simulink model "reg_3_model"  (R2019b)
settings: Solver=VariableStepAuto  StartTime=reg3.ti  StopTime=inf  MaxStep=1e-4  RelTol=1e-9
undefined symbols (not defined in the file): reg3
settings Model: Creator=Charlie  LastModifiedBy=nash

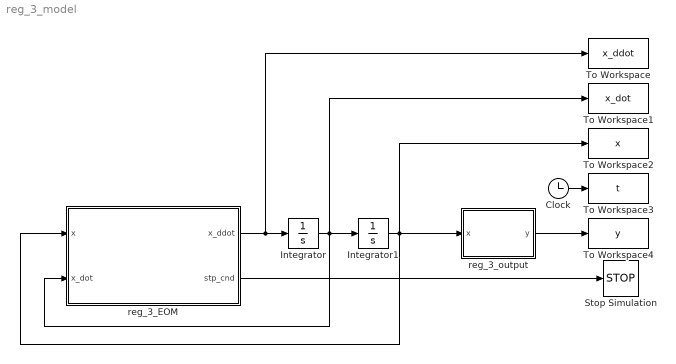
== system reg_3_model ==
  Clock : Clock
  Integrator : Integrator  InitialCondition=reg3.xi_dot
  Integrator1 : Integrator  InitialCondition=reg3.xi
  Stop Simulation : Stop
  To Workspace : ToWorkspace  VariableName=x_ddot  SampleTime=-1
  To Workspace1 : ToWorkspace  VariableName=x_dot  SampleTime=-1
  To Workspace2 : ToWorkspace  VariableName=x  SampleTime=-1
  To Workspace3 : ToWorkspace  VariableName=t  SampleTime=-1
  To Workspace4 : ToWorkspace  VariableName=y  SampleTime=-1
  reg_3_EOM : MATLAB Function  TreatAsAtomicUnit=on
  reg_3_output : MATLAB Function  TreatAsAtomicUnit=on
  wires:
  reg_3_output/1(y) -> To Workspace4/1
  reg_3_EOM/2(stp_cnd) -> Stop Simulation/1
  Clock/1 -> To Workspace3/1
  reg_3_EOM/1(x_ddot) -> To Workspace/1, Integrator/1
  Integrator1/1 -> To Workspace2/1, reg_3_EOM/1(x), reg_3_output/1(x)
  Integrator/1 -> To Workspace1/1, reg_3_EOM/2(x_dot), Integrator1/1

== matlab function reg_3_model/reg_3_output ==
  data: x input; y output; P parameter
%% Regime 3 output equations
%
% This function is responsible for converting the state variables in x to
% the x- and y-coordinates for each point in the mechanism.
%
% This function takes in the following parameters
%   x           The state vector representing the angle of each link
%   P           A MATLAB struct containing all of the constant parameters
% 
% The function returns the following parameters
%   y           The output vector containing the x- and y- coordinates for
%               each point in the mechanism
%
function y  = reg_3_output(x, P)

y = zeros(14,1);

c1 = cos(x(1)); s1 = sin(x(1));
c2 = cos(x(2)); s2 = sin(x(2));
c3 = cos(x(3)); s3 = sin(x(3));

% Point A
y(1)  = 0;                                              % <------
y(2)  = 0;                                              % <------

% Point B
y(3)  = 0;
y(4)  = 0;

% Point C
y(5)  = 0;                                              % <------
y(6)  = 0;                                              % <------

% Point D
y(7)  = 0;                                              % <------
y(8)  = 0;                                              % <------

% Point E
y(9)  = 0;                                              % <------
y(10) = 0;                                              % <------

% Point F
y(11) = 0;                                              % <------
y(12) = 0;                                              % <------

% Point G
y(13) = 0;                                              % <------
y(14) = 0;                                              % <------
% Point D is the origin
y(7)  = 0;
y(8)  = 0;

%% Attempting to use coordinates from Reg 1

% Find point B from point D
y(3)  = y(7) + P.r_BD*c2;
y(4)  = y(8) + P.r_BD*s2;

% Find point C from point D
y(5)  = y(7) + P.r_CD*c2;
y(6)  = y(8) + P.r_CD*s2;

% Find point A from point C
y(1)  = y(5) - P.r_AC*c1;
y(2)  = y(6) - P.r_AC*s1;

% Find point E from point D
y(9)  = y(7) + P.r_DE*c3;
y(10) = y(8) + P.r_DE*s3;

% Find point F from point C
y(11) = y(5) - P.r_CF*c1;
y(12) = y(6) - P.r_CF*s1;

% Find point G
y(13) = y(7) + P.r_DG*c2;
y(14) = y(8) + P.r_DG*s2;

== matlab function reg_3_model/reg_3_EOM ==
  data: x input; x_dot input; x_ddot output; stp_cnd output; P parameter
% Regime 3 equations of motion
%
% This function is responsible for determining the time rate-of-change of
% the state vector representing the angle of each link making up the
% walking arm trebuchet during Regime 3.
%
% Regime 3 is the swinging regime in which all three links move with
% independant velocities.
%
% This function takes in the following parameters
%   x           The state vector representing the angle of each link
%   x_dot       The velocity vector representing the angular velocity of
%               each link.
%   P           A MATLAB struct containing all of the constant parameters
% 
% The function returns the following parameters
%   x_ddot      The acceleration vector representing the angular
%               acceleration of each link.
%   stp_cnd     The stop condition for the simulation. Turns true when
%               the projectile releases from the sling.
%
function [x_ddot, stp_cnd] = reg_3_EOM(x, x_dot, P)

% First, all the angles in the state vector are used to define the sin and
% cos terms needed below.
c1 = cos(x(1)); s1 = sin(x(1)); thd1 = x_dot(1);
c2 = cos(x(2)); s2 = sin(x(2)); thd2 = x_dot(2);
c3 = cos(x(3)); s3 = sin(x(3)); thd3 = x_dot(3);

% Next, the matrix B is defined. This is the same B matrix used in Regime
% 2.
B = [   1           0           0                       
        0           1           0                       
        0           0           1                       
        -P.r_AF*s1  0           0                       
        P.r_AF*s1   0           0                       
        -P.r_AC*s1  -P.r_CG*c2  0                       
        P.r_AC*c1   -P.r_CG*s2  0                       
        -P.r_AC*s1  P.r_CD*c2   -P.r_DE*c3                       
        P.r_AC*c1   P.r_CD*s2   -P.r_DE*s3 ];                    

% Then, the vector b is defined. This vector contains the left over terms
% not accounted for by the B matrix.
b = [   0
        0
        0
        -P.r_AF*c1*thd1^2
        -P.r_AF*s1*thd1^2
        -P.r_AC*c1*thd1^2 + P.r_CG*s2*thd2^2
        -P.r_AC*s1*thd1^2 - P.r_CG*c2*thd2^2
        -P.r_AC*c1*thd1^2 - P.r_CD*s2*thd2^2 + P.r_DE*s3*thd3^2
        -P.r_AC*s1*thd1^2 + P.r_CD*c2*thd2^2 - P.r_DE*c1*thd3^2];

% Then, the matrix M is defined. This matrix combines all of the angular
% and linear accelerations for the "I alpha + r x ma" side of Euler's law.
M = zeros(3,9);
% Row 1 (sum of moments about point A)
M(1,1) =  P.I_1;
M(1,2) =  P.I_2;
M(1,4) = -P.m_1*(-P.r_CF*s1 + P.r_CD*s2);
M(1,5) =  P.m_1*(-P.r_CF*c1 + P.r_CD*c2);
M(1,6) = -P.m_2*(P.r_DG*s2);
M(1,7) =  P.m_2*(P.r_DG*c2);
M(1,8) = -P.m_3*(P.r_DE*s3);
M(1,9) =  P.m_3*(P.r_DE*c3);
% Row 2 (alpha1 = alpha2)
M(2,1) =  1;
M(2,2) = -1;
% Row 3 (alpha1 = alpha3)
M(3,1) =  1;
M(3,3) = -1;
% Then, the vector g is defined. This vector represents all the external
% forces causing moments during the falling regime.
g = [   -P.m_1*P.g                                              
        -P.m_2*P.g                                               
        -P.m_3*P.g ];                                           

% Finally, the acceleration vector is found
x_ddot = (M*B)\(g-M*b);

% The stop condition becomes true when the angle between link 2 and link 3 
% exceeds the selected release angle.
stp_cnd = true;
